simulink model "PILComparison"  (R2014b)
settings: Solver=ode3  StartTime=0.0  StopTime=20  RelTol=1e-3
libraries: LegIK x6, MainController x1, Coord_BodyToLeg x1, TriggerSystem x1, pil_lib x1
Description:
  | Software-in-the-Loop Code Verification
settings Model: ModifiedByFormat=The MathWorks Inc.  ExtModeLogAll=off  ExtModeAutoUpdateStatusClock=off  Creator=The MathWorks Inc.  LastModifiedBy=The MathWorks Inc.
settings DataIOCC: LimitDataPoints=off  SignalLoggingSaveFormat=ModelDataLogs  SignalLogging=off  ReturnWorkspaceOutputs=on  SignalLoggingName=sigsOut  ReturnWorkspaceOutputsName=PCvsBBB
settings OptimizationCC: InlineParams=on  UseDivisionForNetSlopeComputation=UseDivisionForReciprocalsOfIntegersOnly  InlineInvariantSignals=on  EnhancedBackFolding=on  BooleansAsBitfields=on  PassReuseOutputArgsAs=Individual arguments  ExpressionDepthLimit=2147483647  StateBitsets=on  DataBitsets=on  UseTempVars=on  ZeroExternalMemoryAtStartup=off  ZeroInternalMemoryAtStartup=off  NoFixptDivByZeroProtection=on  EfficientFloat2IntCast=on  OptimizeModelRefInitCode=on  LifeSpan=1  MaxStackSize=64
settings DebuggingCC: CheckExecutionContextPreStartOutputMsg=on  CheckExecutionContextRuntimeOutputMsg=on  SolverPrmCheckMsg=none  FcnCallInpInsideContextMsg=UseLocalSettings  UnconnectedLineMsg=none  BusObjectLabelMismatch=error  StateNameClashWarn=warning  StrictBusMsg=ErrorOnBusTreatedAsVector
settings HardwareCC: ProdLargestAtomicInteger=Long  ProdLargestAtomicFloat=Double  ProdEndianess=LittleEndian  ProdHWDeviceType=ARM Compatible->ARM Cortex  TargetLongLongMode=on  TargetEndianess=LittleEndian  TargetHWDeviceType=Generic->MATLAB Host Computer
settings RTWCC: SystemTargetFile=ert.tlc  TemplateMakefile=ert_default_tmf  Description=Embedded Coder  GenerateReport=on  RTWVerbose=off  ProcessScript=ert_make_rtw_hook  Toolchain=Linaro Toolchain v4.8  IncludeHyperlinkInReport=on  PortableWordSizes=on  CreateSILPILBlock=PIL  CodeExecutionProfiling=on  CodeProfilingInstrumentation=on  GenerateTraceInfo=on  GenerateTraceReport=on  GenerateTraceReportSl=on  GenerateTraceReportSf=on  GenerateTraceReportEml=on  GenerateCodeMetricsReport=on
settings CodeAppCC: ForceParamTrailComments=on  IgnoreCustomStorageClasses=off  IgnoreTestpoints=on  SimulinkDataObjDesc=on  CustomSymbolStrGlobalVar=rt$N$M  CustomSymbolStrType=$N$M  CustomSymbolStrFcn=$N$M$F  CustomSymbolStrMacro=$N$M  InsertBlockDesc=on  InternalIdentifier=Classic
settings ERTTargetCC: UtilityFuncGeneration=Shared location  CombineSignalStateStructs=on  SupportNonFinite=off  SupportComplex=off  SupportContinuousTime=on  SupportVariableSizeSignals=on  InlinedParameterPlacement=NonHierarchical  ERTFilePackagingFormat=CompactWithDataFile

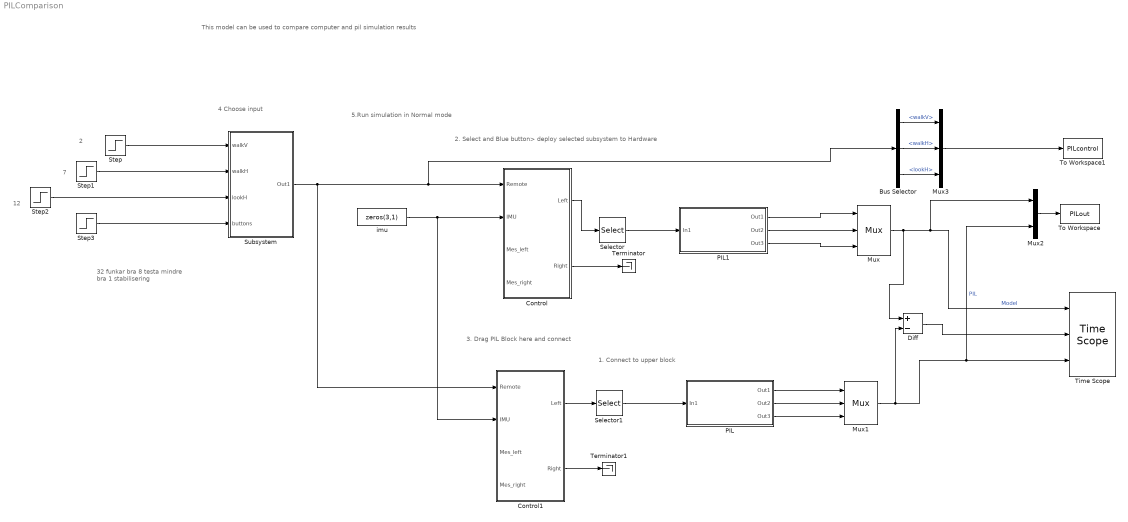
== system PILComparison ==
  note: 12
  note: 7
  note: 2
  note: 4 Choose input
  note: 5.Run simulation in Normal mode
  note: 2. Select and Blue button> deploy selected subsystem to Hardware
  note: 1. Connect to upper block
  note: 3. Drag PIL Block here
      | and connect
  note: This model can be used to compare computer and pil simulation results
  note: 32 funkar bra
      | 8 testa mindre bra
      | 1 stabilisering
  Bus Selector : BusSelector  OutputSignals=walkV,walkH,lookH
  Control : Subsystem  TreatAsAtomicUnit=on
  Control1 : Subsystem  DialogController=pil_create_dialog  LoadFcn=|
      | try
      |    if ~strcmp(rtw.pil.SILPILInterface.getPILVersion, '6.7 (R2014b)_12')
      |       set_param(gcb, 'DialogController', '');
      |       set_param(gcb, 'DialogControllerArgs', '');
      |    end
      | catch e
      |       set_param(gcb, 'DialogController', '');
      |       set_param(gcb, 'DialogControllerArgs', '');
      | end
      mask help: PIL:pil:XILBlockMaskDesc
      mask Display: disp('PIL');
  Diff : Sum  Inputs=+-
  Mux : Mux  Inputs=3
      settings: DisplayOption=signals
  Mux1 : Mux  Inputs=3
      settings: DisplayOption=signals
  Mux2 : Mux  Inputs=2
  Mux3 : Mux  Inputs=3
  PIL : Subsystem
  PIL1 : Subsystem
  Selector : Selector  IndexMode=Zero-based  InputPortWidth=3  IndexOptions=Starting index (dialog)  Indices=0
  Selector1 : Selector  IndexMode=Zero-based  InputPortWidth=3  IndexOptions=Starting index (dialog)  Indices=0
  Step : Step  Time=2  After=50  SampleTime=0.0125
  Step1 : Step  Time=7  After=25  SampleTime=0.0125
  Step2 : Step  Time=12  After=60  SampleTime=0.0125
  Step3 : Step  Time=10  After=0  SampleTime=0.0125
  Subsystem : Subsystem
  Terminator : Terminator
  Terminator1 : Terminator
  Time Scope : TimeScope  ExtModeUploadOption=log  DefaultConfigurationName=spbscopes.TimeScopeBlockCfg  NumInputPorts=3
  To Workspace : ToWorkspace  VariableName=PILout  SaveFormat=Structure With Time  SampleTime=-1
      settings: Save2DSignal=2-D array (concatenate along first dimension)
  To Workspace1 : ToWorkspace  VariableName=PILcontrol  SaveFormat=Structure With Time  SampleTime=-1
  imu : Constant  Value=zeros(3,1)  OutDataTypeStr=double  SampleTime=0.0125
  wires:
  imu/1 -> Control1/2(IMU), Control/2(IMU)
  Mux/1 -> Diff/1, Mux2/1, Time Scope/1  "Model"
  Selector/1 -> PIL1/1(In1)
  PIL1/1(Out1) -> Mux/1
  PIL1/2(Out2) -> Mux/2
  PIL1/3(Out3) -> Mux/3
  PIL/1(Out1) -> Mux1/1
  PIL/2(Out2) -> Mux1/2
  PIL/3(Out3) -> Mux1/3
  Selector1/1 -> PIL/1(In1)
  Mux1/1 -> Diff/2, Mux2/2, Time Scope/3  "PIL"
  Diff/1 -> Time Scope/2
  Step/1 -> Subsystem/1(walkV)
  Step1/1 -> Subsystem/2(walkH)
  Step2/1 -> Subsystem/3(lookH)
  Step3/1 -> Subsystem/4(buttons)
  Mux2/1 -> To Workspace/1
  Subsystem/1(Out1) -> Control1/1(Remote), Control/1(Remote), Bus Selector/1
  Bus Selector/1 -> Mux3/1  "<walkV>"
  Bus Selector/2 -> Mux3/2  "<walkH>"
  Bus Selector/3 -> Mux3/3  "<lookH>"
  Mux3/1 -> To Workspace1/1
  Control1/2(Right) -> Terminator1/1
  Control/1(Left) -> Selector/1
  Control/2(Right) -> Terminator/1
  Control1/1(Left) -> Selector1/1

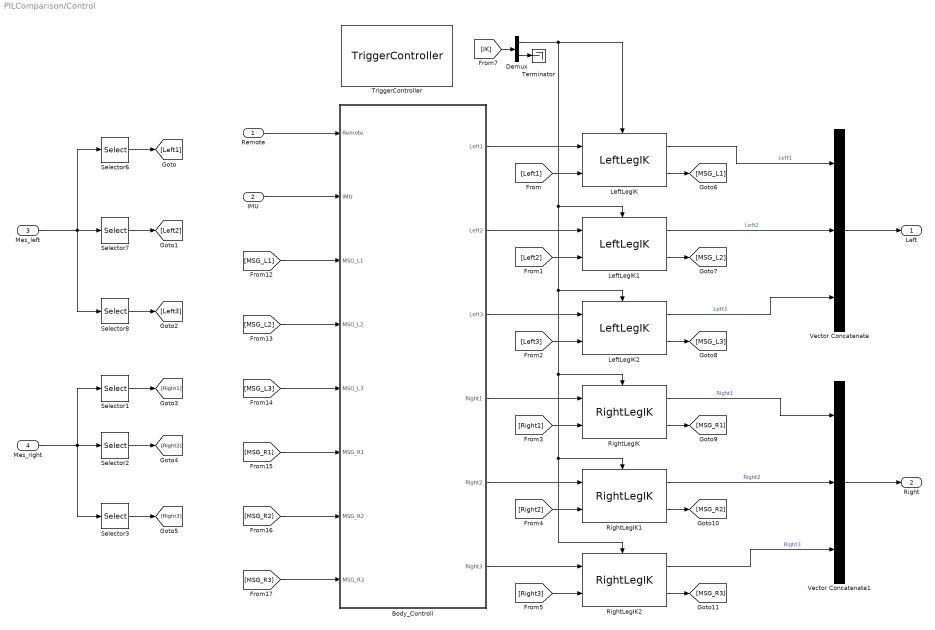
== system PILComparison/Control ==
  Remote : Inport  OutDataTypeStr=Bus: Command
  IMU : Inport  Port=2
  Mes_left : Inport  Port=3  OutDataTypeStr=Bus: Leg_mes
  Mes_right : Inport  Port=4  OutDataTypeStr=Bus: Leg_mes
  Body_Controll : Subsystem
  Demux : Demux  Outputs=2
  LeftLegIK : LegIK/LeftLegIK  ID1=1  ID2=3  ID3=5
  LeftLegIK1 : LegIK/LeftLegIK  ID1=13  ID2=15  ID3=17
  LeftLegIK2 : LegIK/LeftLegIK  ID1=7  ID2=9  ID3=11
  RightLegIK : LegIK/RightLegIK  ID1=2  ID2=4  ID3=6
  RightLegIK1 : LegIK/RightLegIK  ID1=14  ID2=16  ID3=18
  RightLegIK2 : LegIK/RightLegIK  ID1=8  ID2=10  ID3=12
  Selector1 : Selector  IndexMode=Zero-based  InputPortWidth=3  Indices=0
  Selector2 : Selector  IndexMode=Zero-based  InputPortWidth=3
  Selector3 : Selector  IndexMode=Zero-based  InputPortWidth=3  Indices=2
  Selector6 : Selector  IndexMode=Zero-based  InputPortWidth=3  Indices=0
  Selector7 : Selector  IndexMode=Zero-based  InputPortWidth=3
  Selector8 : Selector  IndexMode=Zero-based  InputPortWidth=3  Indices=2
  Terminator : Terminator
  TriggerController : TriggerSystem/TriggerController  f=40
  Vector Concatenate : Concatenate  NumInputs=3  ConcatenateDimension=2
  Vector Concatenate1 : Concatenate  NumInputs=3  ConcatenateDimension=2
  Left : Outport  OutDataTypeStr=Bus: Leg_ref
  Right : Outport  Port=2  OutDataTypeStr=Bus: Leg_ref
  wires:
  Body_Controll/2(Left2) -> LeftLegIK1/1
  Body_Controll/1(Left1) -> LeftLegIK/1
  Body_Controll/3(Left3) -> LeftLegIK2/1
  Body_Controll/5(Right2) -> RightLegIK1/1
  Body_Controll/4(Right1) -> RightLegIK/1
  Body_Controll/6(Right3) -> RightLegIK2/1
  Remote/1 -> Body_Controll/1(Remote)
  [Left3] -> LeftLegIK2/2
  [Right1] -> RightLegIK/2
  RightLegIK/2 -> [MSG_R1]
  [MSG_R3] -> Body_Controll/8(MSG_R3)
  [MSG_R2] -> Body_Controll/7(MSG_R2)
  [MSG_R1] -> Body_Controll/6(MSG_R1)
  [MSG_L3] -> Body_Controll/5(MSG_L3)
  [MSG_L2] -> Body_Controll/4(MSG_L2)
  [MSG_L1] -> Body_Controll/3(MSG_L1)
  RightLegIK2/2 -> [MSG_R3]
  LeftLegIK2/2 -> [MSG_L3]
  RightLegIK1/2 -> [MSG_R2]
  LeftLegIK1/2 -> [MSG_L2]
  LeftLegIK/2 -> [MSG_L1]
  [Right2] -> RightLegIK1/2
  IMU/1 -> Body_Controll/2(IMU)
  [Right3] -> RightLegIK2/2
  [Left1] -> LeftLegIK/2
  [Left2] -> LeftLegIK1/2
  LeftLegIK2/1 -> Vector Concatenate/3  "Left3"
  LeftLegIK1/1 -> Vector Concatenate/2  "Left2"
  LeftLegIK/1 -> Vector Concatenate/1  "Left1"
  Vector Concatenate/1 -> Left/1
  RightLegIK/1 -> Vector Concatenate1/1  "Right1"
  RightLegIK1/1 -> Vector Concatenate1/2  "Right2"
  RightLegIK2/1 -> Vector Concatenate1/3  "Right3"
  Vector Concatenate1/1 -> Right/1
  Mes_left/1 -> Selector6/1, Selector7/1, Selector8/1
  Selector6/1 -> [Left1]
  Selector7/1 -> [Left2]
  Selector8/1 -> [Left3]
  Mes_right/1 -> Selector3/1, Selector2/1, Selector1/1
  Selector1/1 -> [Right1]
  Selector2/1 -> [Right2]
  Selector3/1 -> [Right3]
  Demux/1 -> RightLegIK1/Trigger, RightLegIK2/Trigger, RightLegIK/Trigger, LeftLegIK2/Trigger, LeftLegIK1/Trigger, LeftLegIK/Trigger
  [IK] -> Demux/1
  Demux/2 -> Terminator/1

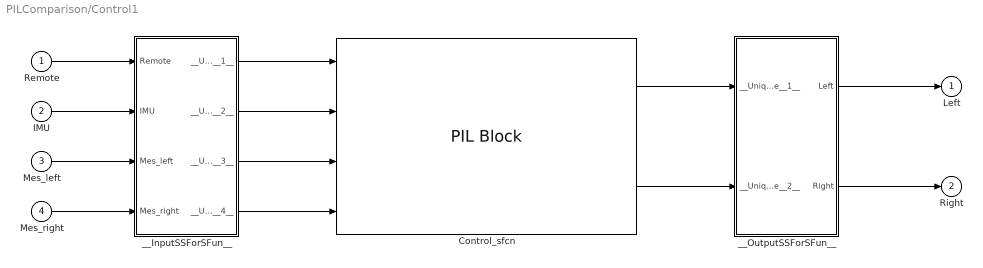
== system PILComparison/Control1 ==
  Remote : Inport  OutDataTypeStr=Bus: Command
  IMU : Inport  Port=2
  Mes_left : Inport  Port=3  OutDataTypeStr=Bus: Leg_mes  BusOutputAsStruct=on
  Mes_right : Inport  Port=4  OutDataTypeStr=Bus: Leg_mes  BusOutputAsStruct=on
  Control_sfcn : pil_lib/PIL Block  SimulationMode=PIL  IsTopModelPIL=off  CodeDir=C:\Users\Sebastian\Hexapod\CodeGeneration\Control_ert_rtw  ConfigName=BeagleBone Black
  __InputSSForSFun__ : Subsystem
  __OutputSSForSFun__ : Subsystem
  Left : Outport  OutDataTypeStr=Bus: Leg_ref  SampleTime=[0.012500000000000001 0]  BusOutputAsStruct=on
  Right : Outport  Port=2  OutDataTypeStr=Bus: Leg_ref  SampleTime=[0.012500000000000001 0]  BusOutputAsStruct=on
  wires:
  __OutputSSForSFun__/2(Right) -> Right/1
  __OutputSSForSFun__/1(Left) -> Left/1
  Control_sfcn/2 -> __OutputSSForSFun__/2(__UniqueInportName__2__)
  Control_sfcn/1 -> __OutputSSForSFun__/1(__UniqueInportName__1__)
  __InputSSForSFun__/4(__UniqueOutportName__4__) -> Control_sfcn/4
  __InputSSForSFun__/3(__UniqueOutportName__3__) -> Control_sfcn/3
  __InputSSForSFun__/2(__UniqueOutportName__2__) -> Control_sfcn/2
  __InputSSForSFun__/1(__UniqueOutportName__1__) -> Control_sfcn/1
  Mes_right/1 -> __InputSSForSFun__/4(Mes_right)
  Mes_left/1 -> __InputSSForSFun__/3(Mes_left)
  IMU/1 -> __InputSSForSFun__/2(IMU)
  Remote/1 -> __InputSSForSFun__/1(Remote)

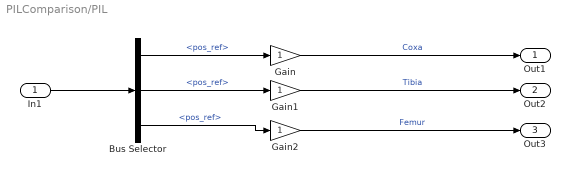
== system PILComparison/PIL ==
  In1 : Inport
  Bus Selector : BusSelector  OutputSignals=Servo1.pos_ref,Servo2.pos_ref,Servo3.pos_ref
  Gain : Gain
  Gain1 : Gain
  Gain2 : Gain
  Out1 : Outport
  Out2 : Outport  Port=2
  Out3 : Outport  Port=3
  wires:
  Gain2/1 -> Out3/1  "Femur"
  Gain1/1 -> Out2/1  "Tibia"
  Bus Selector/3 -> Gain2/1  "<pos_ref>"
  Bus Selector/1 -> Gain/1  "<pos_ref>"
  In1/1 -> Bus Selector/1
  Bus Selector/2 -> Gain1/1  "<pos_ref>"
  Gain/1 -> Out1/1  "Coxa"

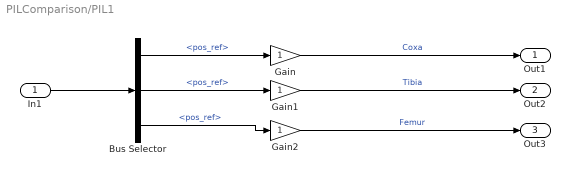
== system PILComparison/PIL1 ==
  In1 : Inport
  Bus Selector : BusSelector  OutputSignals=Servo1.pos_ref,Servo2.pos_ref,Servo3.pos_ref
  Gain : Gain
  Gain1 : Gain
  Gain2 : Gain
  Out1 : Outport
  Out2 : Outport  Port=2
  Out3 : Outport  Port=3
  wires:
  Gain2/1 -> Out3/1  "Femur"
  Gain1/1 -> Out2/1  "Tibia"
  Bus Selector/3 -> Gain2/1  "<pos_ref>"
  Bus Selector/1 -> Gain/1  "<pos_ref>"
  In1/1 -> Bus Selector/1
  Bus Selector/2 -> Gain1/1  "<pos_ref>"
  Gain/1 -> Out1/1  "Coxa"

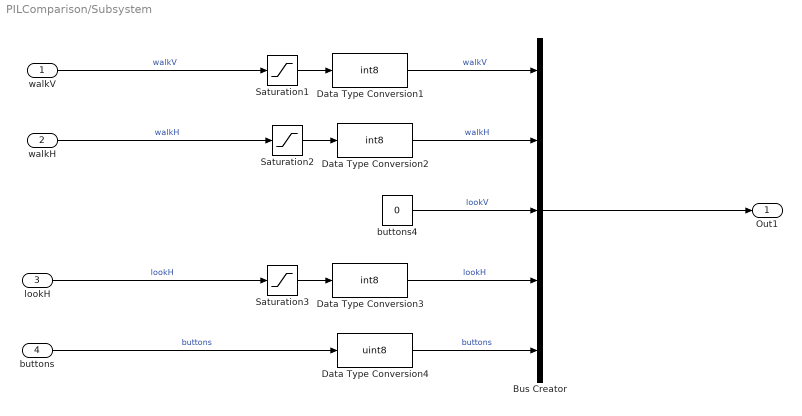
== system PILComparison/Subsystem ==
  walkV : Inport
  walkH : Inport  Port=2
  lookH : Inport  Port=3
  buttons : Inport  Port=4
  Bus Creator : BusCreator  Inputs=5  OutDataTypeStr=Bus: Command
  Data Type Conversion1 : DataTypeConversion  OutDataTypeStr=int8
  Data Type Conversion2 : DataTypeConversion  OutDataTypeStr=int8
  Data Type Conversion3 : DataTypeConversion  OutDataTypeStr=int8
  Data Type Conversion4 : DataTypeConversion  OutDataTypeStr=uint8
  Saturation1 : Saturate  UpperLimit=50  LowerLimit=-30
  Saturation2 : Saturate  UpperLimit=50  LowerLimit=-30
  Saturation3 : Saturate  UpperLimit=50  LowerLimit=-50
  buttons4 : Constant  Value=0  OutDataTypeStr=int8  SampleTime=-1
  Out1 : Outport
  wires:
  walkH/1 -> Saturation2/1  "walkH"
  Saturation2/1 -> Data Type Conversion2/1
  walkV/1 -> Saturation1/1  "walkV"
  Data Type Conversion1/1 -> Bus Creator/1  "walkV"
  Saturation1/1 -> Data Type Conversion1/1
  Data Type Conversion2/1 -> Bus Creator/2  "walkH"
  Data Type Conversion3/1 -> Bus Creator/4  "lookH"
  Bus Creator/1 -> Out1/1
  buttons4/1 -> Bus Creator/3  "lookV"
  lookH/1 -> Saturation3/1  "lookH"
  Saturation3/1 -> Data Type Conversion3/1
  buttons/1 -> Data Type Conversion4/1  "buttons"
  Data Type Conversion4/1 -> Bus Creator/5  "buttons"

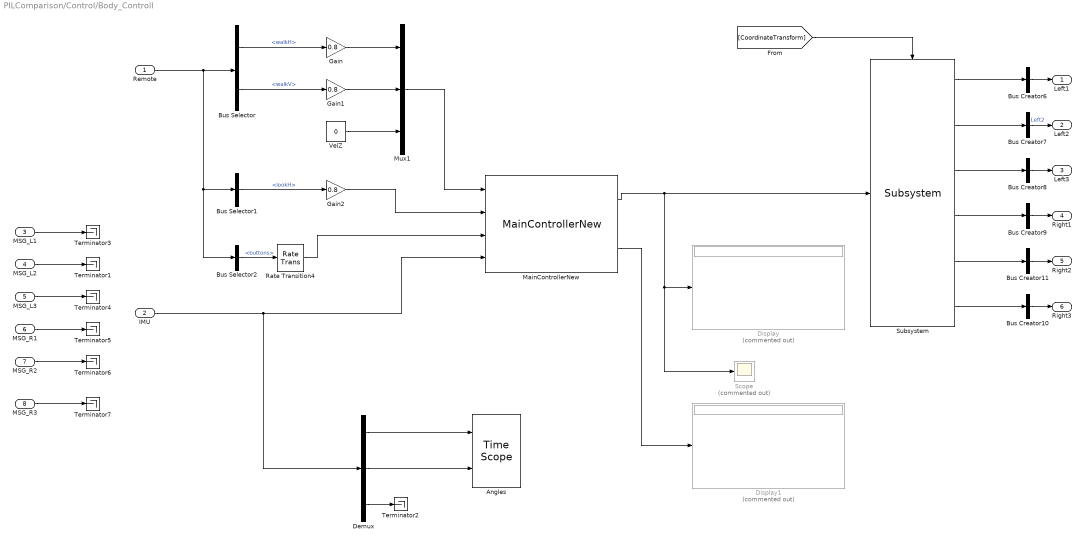
== system PILComparison/Control/Body_Controll ==
  Remote : Inport  OutDataTypeStr=Bus: Command
  IMU : Inport  Port=2
  MSG_L1 : Inport  Port=3
  MSG_L2 : Inport  Port=4
  MSG_L3 : Inport  Port=5
  MSG_R1 : Inport  Port=6
  MSG_R2 : Inport  Port=7
  MSG_R3 : Inport  Port=8
  Angles : TimeScope  DefaultConfigurationName=spbscopes.TimeScopeBlockCfg  NumInputPorts=2
  Bus Creator{6..11} (6 alike) : BusCreator  Inputs=1  OutDataTypeStr=Bus: Leg_data
      settings: InheritFromInputs=off
  Bus Selector : BusSelector  OutputSignals=walkH,walkV
  Bus Selector1 : BusSelector  OutputSignals=lookH
  Bus Selector2 : BusSelector  OutputSignals=buttons
  Demux : Demux  Outputs=3
  Display : Display  Commented=on
  Display1 : Display  Commented=on
  Gain : Gain  Gain=0.8  OutDataTypeStr=double
  Gain1 : Gain  Gain=0.8  OutDataTypeStr=double
  Gain2 : Gain  Gain=0.8  OutDataTypeStr=double
  MainControllerNew : MainController/MainControllerNew
  Mux1 : Mux  Inputs=3
  Rate Transition4 : RateTransition  Deterministic=off  OutPortSampleTime=0.0125
  Scope : Scope  Commented=on
      settings: YMin=-300  YMax=400  SaveName=ScopeData5
  Subsystem : Coord_BodyToLeg/Subsystem
  Terminator{1..7} (7 alike) : Terminator
  VelZ : Constant  Value=0  OutDataTypeStr=double  SampleTime=0.0125
  Left1 : Outport  OutDataTypeStr=Bus: Leg_data
  Left2 : Outport  Port=2  OutDataTypeStr=Bus: Leg_data
  Left3 : Outport  Port=3  OutDataTypeStr=Bus: Leg_data
  Right1 : Outport  Port=4  OutDataTypeStr=Bus: Leg_data
  Right2 : Outport  Port=5  OutDataTypeStr=Bus: Leg_data
  Right3 : Outport  Port=6  OutDataTypeStr=Bus: Leg_data
  wires:
  MSG_R3/1 -> Terminator7/1
  MSG_L1/1 -> Terminator3/1
  MSG_L2/1 -> Terminator1/1
  MSG_L3/1 -> Terminator4/1
  MSG_R1/1 -> Terminator5/1
  MSG_R2/1 -> Terminator6/1
  Subsystem/1 -> Bus Creator6/1
  Subsystem/2 -> Bus Creator7/1
  Subsystem/3 -> Bus Creator8/1
  Subsystem/4 -> Bus Creator9/1
  Subsystem/5 -> Bus Creator11/1
  Subsystem/6 -> Bus Creator10/1
  Bus Creator10/1 -> Right3/1
  Bus Creator11/1 -> Right2/1
  Bus Creator9/1 -> Right1/1
  Bus Creator8/1 -> Left3/1
  Bus Creator7/1 -> Left2/1  "Left2"
  Bus Creator6/1 -> Left1/1
  VelZ/1 -> Mux1/3
  Mux1/1 -> MainControllerNew/1
  MainControllerNew/1 -> Subsystem/1, Scope/1, Display/1
  MainControllerNew/2 -> Display1/1
  Bus Selector/1 -> Gain/1  "<walkH>"
  Bus Selector/2 -> Gain1/1  "<walkV>"
  Gain/1 -> Mux1/1
  Bus Selector1/1 -> Gain2/1  "<lookH>"
  Gain1/1 -> Mux1/2
  Remote/1 -> Bus Selector/1, Bus Selector2/1, Bus Selector1/1
  Bus Selector2/1 -> Rate Transition4/1  "<buttons>"
  Demux/1 -> Angles/1
  Demux/2 -> Angles/2
  [CoordinateTransform] -> Subsystem/Trigger
  Gain2/1 -> MainControllerNew/2
  Demux/3 -> Terminator2/1
  Rate Transition4/1 -> MainControllerNew/3
  IMU/1 -> MainControllerNew/4, Demux/1

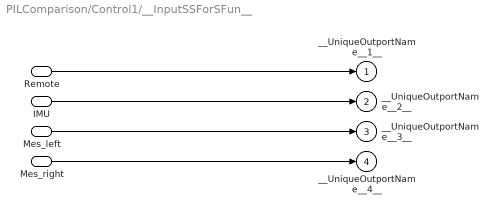
== system PILComparison/Control1/__InputSSForSFun__ ==
  Remote : Inport  OutDataTypeStr=Bus: Command
  IMU : Inport  Port=2
  Mes_left : Inport  Port=3  OutDataTypeStr=Bus: Leg_mes  BusOutputAsStruct=on
  Mes_right : Inport  Port=4  OutDataTypeStr=Bus: Leg_mes  BusOutputAsStruct=on
  __UniqueOutportName__1__ : Outport
  __UniqueOutportName__2__ : Outport  Port=2
  __UniqueOutportName__3__ : Outport  Port=3
  __UniqueOutportName__4__ : Outport  Port=4
  wires:
  Mes_right/1 -> __UniqueOutportName__4__/1
  Mes_left/1 -> __UniqueOutportName__3__/1
  IMU/1 -> __UniqueOutportName__2__/1
  Remote/1 -> __UniqueOutportName__1__/1

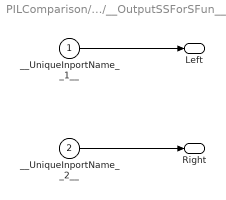
== system PILComparison/Control1/__OutputSSForSFun__ ==
  __UniqueInportName__1__ : Inport
  __UniqueInportName__2__ : Inport  Port=2
  Left : Outport  OutDataTypeStr=Bus: Leg_ref  SampleTime=[0.012500000000000001 0]  BusOutputAsStruct=on
  Right : Outport  Port=2  OutDataTypeStr=Bus: Leg_ref  SampleTime=[0.012500000000000001 0]  BusOutputAsStruct=on
  wires:
  __UniqueInportName__2__/1 -> Right/1
  __UniqueInportName__1__/1 -> Left/1
